simulink model "path2_2021a"  (R2021a)
settings: Solver=VariableStepAuto  StartTime=0.0  StopTime=10.0  RelTol=1e-3
undefined symbols (not defined in the file or in its folder): DiscIntNeverNeededParam
libraries: simulink x1
settings Model: Creator=jiaweichen  LastModifiedBy=jiaweichen
settings DebuggingCC: UnconnectedInputMsg=none  UnconnectedOutputMsg=none  UnconnectedLineMsg=none
settings ModelReferenceCC: EnableRefExpFcnMdlSchedulingChecks=off
settings RTWCC: Description=Generic Real-Time Target  DLArmComputeVersion=20.02.1

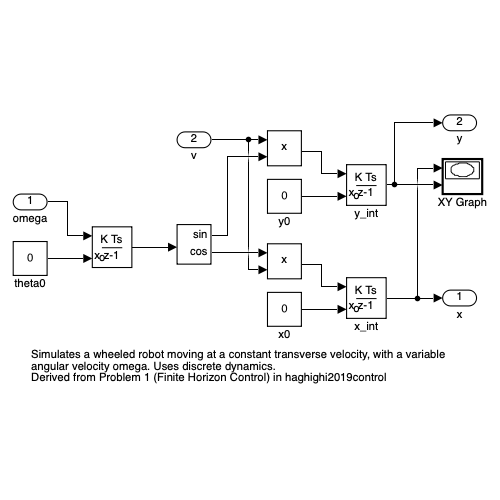
[thumbnail: Simulink's stored preview of the top-level diagram]
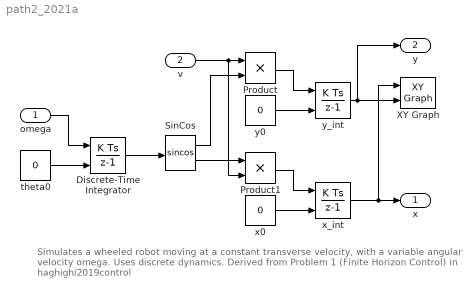
== system path2_2021a ==
  note: Simulates a wheeled robot moving at a constant transverse velocity, with a variable angular velocity omega. Uses discrete dynamics.
      | Derived from Problem 1 (Finite Horizon Control) in haghighi2019control
  omega : Inport
  v : Inport  Port=2
  Discrete-Time Integrator : DiscreteIntegrator  InitialConditionSource=external  SampleTime=0.1  ICPrevOutput=DiscIntNeverNeededParam  ICPrevScaledInput=DiscIntNeverNeededParam
  Product : Product
  Product1 : Product
  SinCos : Trigonometry  Operator=sincos
  XY Graph : simulink/Sinks/XY Graph  xmin=-1  xmax=1  ymin=-1  ymax=1  st=-1
  theta0 : Constant  Value=0
  x0 : Constant  Value=0
  x_int : DiscreteIntegrator  InitialConditionSource=external  SampleTime=0.1  ICPrevOutput=DiscIntNeverNeededParam  ICPrevScaledInput=DiscIntNeverNeededParam
  y0 : Constant  Value=0
  y_int : DiscreteIntegrator  InitialConditionSource=external  SampleTime=0.1  ICPrevOutput=DiscIntNeverNeededParam  ICPrevScaledInput=DiscIntNeverNeededParam
  x : Outport
  y : Outport  Port=2
  wires:
  x_int/1 -> x/1, XY Graph/1
  Discrete-Time Integrator/1 -> SinCos/1
  x0/1 -> x_int/2
  Product/1 -> y_int/1
  y0/1 -> y_int/2
  y_int/1 -> y/1, XY Graph/2
  SinCos/2 -> Product1/1
  SinCos/1 -> Product/2
  v/1 -> Product/1, Product1/2
  Product1/1 -> x_int/1
  theta0/1 -> Discrete-Time Integrator/2
  omega/1 -> Discrete-Time Integrator/1
